simulink subsystem "Pack_Actors_Info"  (R2024a)
settings: Solver=VariableStepAuto  StartTime=0.0  StopTime=10.0  RelTol=1e-3
undefined symbols (not defined in the file): actorsClassID
libraries: simulink x1
settings Model: Creator=L03509110  LastModifiedBy=L03509110

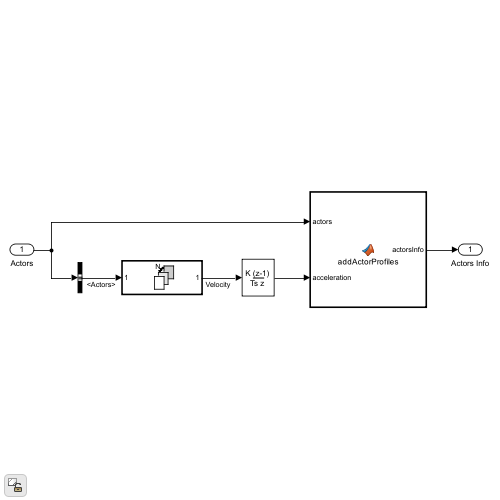
[thumbnail: Simulink's stored preview of the top-level diagram]
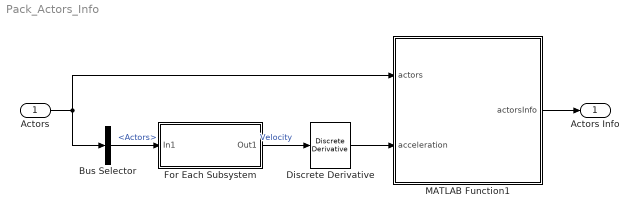
== system Pack_Actors_Info ==
  Actors : Inport
  Bus Selector : BusSelector  OutputSignals=Actors
  Discrete Derivative : simulink/Discrete/Discrete Derivative  gainval=1.0  ICPrevScaledInput=0.0  OutMin=[]  OutMax=[]  OutDataType=fixdt(1, 16)  OutScaling=2^-10  DoSatur=off
  For Each Subsystem : Subsystem  TreatAsAtomicUnit=on
  MATLAB Function1 : MATLAB Function  TreatAsAtomicUnit=on  mask{outputStruct=Simulink.Bus.createMATLABStruct('BusActorsInfo')}
      mask prompts: outputStruct "Output Struct"
  Actors Info : Outport
  wires:
  MATLAB Function1/1(actorsInfo) -> Actors Info/1
  Actors/1 -> MATLAB Function1/1(actors), Bus Selector/1
  Bus Selector/1 -> For Each Subsystem/1(In1)  "<Actors>"
  For Each Subsystem/1(Out1) -> Discrete Derivative/1  "Velocity"
  Discrete Derivative/1 -> MATLAB Function1/2(acceleration)

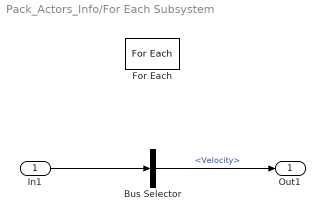
== system Pack_Actors_Info/For Each Subsystem ==
  In1 : Inport  Partition=on  PartitionDimension=1  PartitionWidth=1  PartitionOffset=0
  Bus Selector : BusSelector  OutputSignals=Velocity
  For Each : ForEach  DisableCoverage=on
  Out1 : Outport  ConcatenationDimension=1
  wires:
  Bus Selector/1 -> Out1/1  "<Velocity>"
  In1/1 -> Bus Selector/1

== matlab function Pack_Actors_Info/MATLAB Function1 ==
  data: actors input; acceleration input; actorsInfo output Bus: BusActorsInfo; actorsClassID parameter; outputStruct parameter
function actorsInfo = addActorProfiles(actors,acceleration,actorsClassID,outputStruct) 
    actorsInfo = outputStruct;
    outputStruct.NumActors = actors.NumActors;
    outputStruct.Time      = actors.Time;
    for i = 1:actors.NumActors
        outputStruct.Actors(i).ActorID  = actors.Actors(i).ActorID;
        classId = actorsClassID((actorsClassID(:,1) == actors.Actors(i).ActorID) ,2);
        length  = actorsClassID((actorsClassID(:,1) == actors.Actors(i).ActorID) ,3);
        width   = actorsClassID((actorsClassID(:,1) == actors.Actors(i).ActorID) ,4);
        outputStruct.Actors(i).ClassID  = classId(1);
        outputStruct.Actors(i).Position = actors.Actors(i).Position;
        outputStruct.Actors(i).Velocity = actors.Actors(i).Velocity;
        outputStruct.Actors(i).Acceleration = acceleration(i,:);
        outputStruct.Actors(i).Roll  = actors.Actors(i).Roll;
        outputStruct.Actors(i).Pitch = actors.Actors(i).Pitch;
        outputStruct.Actors(i).Yaw   = actors.Actors(i).Yaw;
        outputStruct.Actors(i).Length   = length(1);
        outputStruct.Actors(i).Width   = width(1);
    end
    actorsInfo = outputStruct;
end
